simulink model "ModeloSK"  (R2022b)
settings: Solver=FixedStepAuto  StartTime=0.0  StopTime=Tsim  FixedStep=Ts  RelTol=1e-3
values from neighbouring files (symbols this model uses):
  K = 0.35    [Sintonizacion.m]
  Kc = (1/(mu*K))*(0.9+mu/12)    (= 4.32212885154)    [Sintonizacion.m]
  t0 = 8.5    [Sintonizacion.m]
  Tau = 13.5    [Sintonizacion.m]
  Ti = t0*((30+3*mu)/(9+20*mu))    (= 12.5531732419)    [Sintonizacion.m]
  X0 = 0.25    [Sintonizacion.m]
settings Model: Creator=auditorio  LastModifiedBy=auditorio

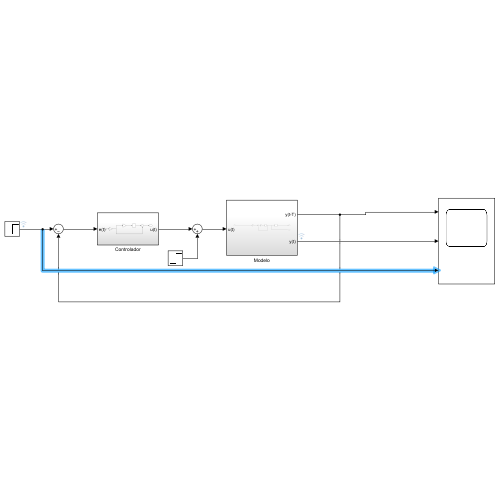
[thumbnail: Simulink's stored preview of the top-level diagram]
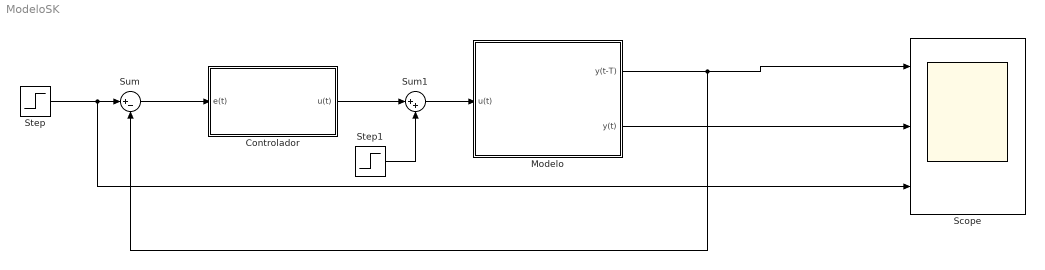
== system ModeloSK ==
  Controlador : Subsystem
  Modelo : Subsystem
  Scope : Scope  NumInputPorts=3
  Step : Step  Time=250  Before=X0  After=0.3  SampleTime=0
  Step1 : Step  Time=500  After=0.01  SampleTime=0
  Sum : Sum  Inputs=|+-
  Sum1 : Sum  Inputs=|++
  wires:
  Modelo/1(y(t-T)) -> Sum/2, Scope/1
  Modelo/2(y(t)) -> Scope/2
  Sum/1 -> Controlador/1(e(t))
  Step/1 -> Scope/3, Sum/1
  Controlador/1(u(t)) -> Sum1/1
  Sum1/1 -> Modelo/1(u(t))
  Step1/1 -> Sum1/2

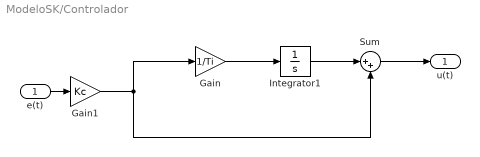
== system ModeloSK/Controlador ==
  e(t) : Inport
  Gain : Gain  Gain=1/Ti
  Gain1 : Gain  Gain=Kc
  Integrator1 : Integrator  InitialCondition=X0/K
  Sum : Sum  Inputs=|++
  u(t) : Outport
  wires:
  Gain1/1 -> Sum/2, Gain/1
  Gain/1 -> Integrator1/1
  Integrator1/1 -> Sum/1
  Sum/1 -> u(t)/1
  e(t)/1 -> Gain1/1

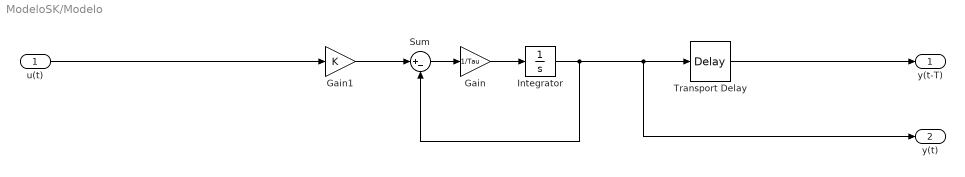
== system ModeloSK/Modelo ==
  u(t) : Inport
  Gain : Gain  Gain=1/Tau
  Gain1 : Gain  Gain=K
  Integrator : Integrator  InitialCondition=X0
  Sum : Sum  Inputs=|+-
  Transport Delay : TransportDelay  DelayTime=t0  InitialOutput=X0
  y(t-T) : Outport
  y(t) : Outport  Port=2
  wires:
  Integrator/1 -> y(t)/1, Transport Delay/1, Sum/2
  Sum/1 -> Gain/1
  Gain/1 -> Integrator/1
  Gain1/1 -> Sum/1
  Transport Delay/1 -> y(t-T)/1
  u(t)/1 -> Gain1/1
